simulink model "simu"  (R2019b)
settings: Solver=VariableStepAuto  StartTime=0.0  StopTime=5  RelTol=1e-3
values from neighbouring files (symbols this model uses):
  acp = K.A    [P1.m]    (also in P1_modify.m; P2.m)
  ag = [ ... (first row only)    [P2.m]    (also in hmatdemo.m)
  bcp = K.B    [P1.m]    (also in P1_modify.m; P2.m)
  bg = [0     0 ... (first row only)    [P2.m]    (also in hmatdemo.m)
  ccp = K.C    [P1.m]    (also in P1_modify.m; P2.m)
  cg = [0     1     0     0     0     0 ... (first row only)    [P2.m]    (also in hmatdemo.m)
  dcp = K.D    [P1.m]    (also in P1_modify.m; P2.m)
  dg = [0     0 ... (first row only)    [P2.m]    (also in hmatdemo.m)
settings Model: Creator=miaokeyan  LastModifiedBy=miaokeyan

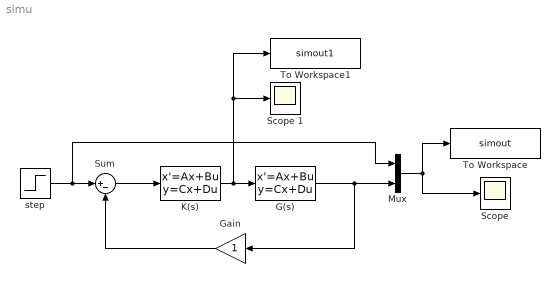
== system simu ==
  G(s) : StateSpace  A=ag  B=bg  C=cg  D=dg  InitialCondition=0
  Gain : Gain
  K(s) : StateSpace  A=acp  B=bcp  C=ccp  D=dcp  InitialCondition=0
  Mux : Mux  Inputs=2
  "Scope " : Scope
  Scope 1 : Scope
  Sum : Sum  Inputs=|+-
  To Workspace : ToWorkspace  VariableName=simout  SaveFormat=Timeseries  SampleTime=-1
  To Workspace1 : ToWorkspace  VariableName=simout1  SaveFormat=Timeseries  SampleTime=-1
  step : Step  Time=0  SampleTime=0
  wires:
  step/1 -> Mux/1, Sum/1
  Sum/1 -> K(s)/1
  Gain/1 -> Sum/2
  Mux/1 -> "Scope "/1, To Workspace/1
  K(s)/1 -> To Workspace1/1, Scope 1/1, G(s)/1
  G(s)/1 -> Mux/2, Gain/1
